simulink subsystem "PMSM_Controller"  (R2021b)
settings: Solver=VariableStepAuto  StartTime=0.0  StopTime=10.0  RelTol=1e-3
model mask{ControllerParameters=0}
  mask prompts: ControllerParameters "Controller Parameters (struct)"
undefined symbols (not defined in the file): denZC_id, denZC_iq, denZC_w, ee_sli_rtmsupport, gcbh, numZC_id, numZC_iq, numZC_w, PowSupplyParams
libraries: eeDiscretePi x3, slctrlblks x2, eeTransforms x2, eeDqVoltageLimiter x1, eePmsmCurrentReferenceGen x1, simulink x1, eePwmGeneratorTwoLevel x1
Description:
  | PMSM Controller Subsystem Reference.
  | Copyright 2021 The MathWorks, Inc.
settings Model: Creator=agonzale  LastModifiedBy=agonzale

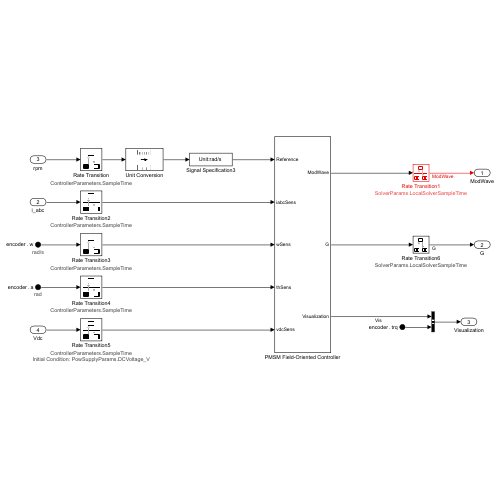
[thumbnail: Simulink's stored preview of the top-level diagram]
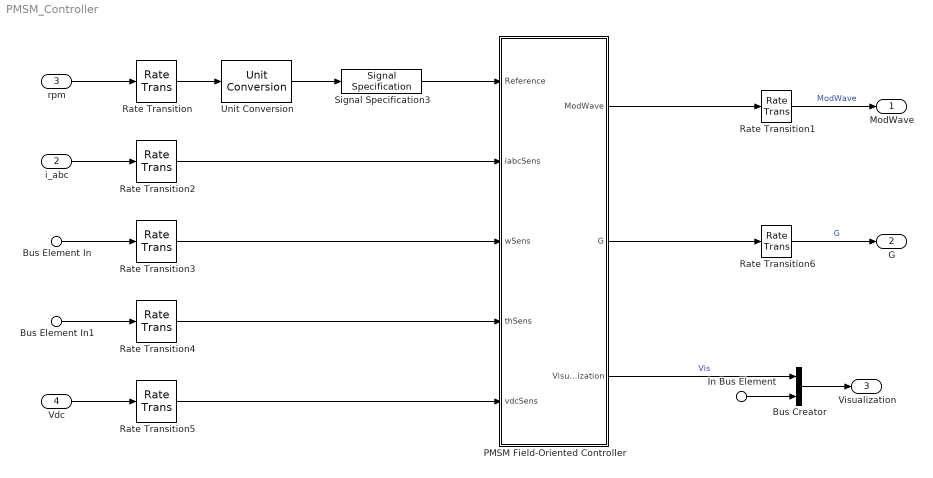
== system PMSM_Controller ==
  Bus Element In : Inport  PortName=encoder  Element=w
      settings: AttributesFormatString=%<Unit>
  Bus Element In1 : Inport  PortName=encoder  Element=a
      settings: AttributesFormatString=%<Unit>
  In Bus Element : Inport  PortName=encoder  Element=trq
  i_abc : Inport  Port=2
  rpm : Inport  Port=3  Unit=rpm
  Vdc : Inport  Port=4
  Bus Creator : BusCreator  Inputs=2
  PMSM Field-Oriented Controller : Subsystem  LoadFcn=ee_sli_rtmsupport( 'loadfcn', gcbh );  VariantControl=Estimation  mask(PMSM Field-Oriented Control){winding_type=Wye-wound, CtrlMode=Velocity control, Vnom=ControllerParameters.VdcNominal, Pmax=ControllerParameters.PowMax, Tmax=ControllerParameters.TrqMax, p=ControllerParameters.NumPolePairs, Vdc_on=ControllerParameters.InverterVdcThreshold, Ts=ControllerParameters.FundamentalSampleTime, Tsc=ControllerParameters.SampleTime, CtrlType=PI control, Kp_w=ControllerParameters.OuterLoop.PropGain, Ki_w=ControllerParameters.OuterLoop.IntegGain, Kv_w=1, Kaw_w=ControllerParameters.OuterLoop.AntiWindupIntegGain, RefType=Lookup-table based, rpmVec=ControllerParameters.OuterLoop.RpmVec, TqVec=ControllerParameters.OuterLoop.TrqRefVec, VdcVec=ControllerParameters.OuterLoop.VdcVec, PWMMode=SPWM: sinusoidal PWM, ModFactor=1, idMatrix=ControllerParameters.OuterLoop.iDrefMat, iqMatrix=ControllerParameters.OuterLoop.iQrefMat, psim=1, Ld=0.00024, Lq=0.00029, Rs=1, AxisAlignment=Q-axis, Kp_id=ControllerParameters.InnerLoop.PropGain_iD, Ki_id=ControllerParameters.InnerLoop.IntegGain_iD, Kaw_id=ControllerParameters.InnerLoop.AntiWindupIntegGain_iD, Kp_iq=ControllerParameters.InnerLoop.PropGain_iQ, Ki_iq=ControllerParameters.InnerLoop.IntegGain_iQ, Kaw_iq=ControllerParameters.InnerLoop.AntiWindupIntegGain_iQ, AxisPrio=Q-axis, ActZC=off, ActFF=off, ParamTypeFF=Constant parameters, LdFF=1, LqFF=1, psimFF=1, idVect=[-200, 0, 200], iqVect=[-200, 0, 200], LdMatrix=0.0002 * ones(3, 3), LqMatrix=0.0002 * ones(3, 3), psimMatrix=0.04 * ones(3, 3), CPWMMode=SPWM: sinusoidal PWM, SamplingMode=Natural, fsw=ControllerParameters.InverterSwitchingFrequency}
      mask prompts: winding_type "Winding type"; CtrlMode "physmod:ee:library:comments:control:eePmsmFieldOrientedControl:ControlMode_MP"; Vnom "physmod:ee:library:comments:control:eePmsmFieldOrientedControl:NominalDclinkVoltageV_MP"; Pmax "physmod:ee:library:comments:control:eePmsmFieldOrientedControl:MaximumPowerW_MP"; Tmax "physmod:ee:library:comments:control:eePmsmFieldOrientedControl:MaximumTorqueNm_MP"; p "physmod:ee:library:comments:control:eePmsmFieldOrientedControl:NumberOfRotorPolePairs_MP"; Vdc_on "physmod:ee:library:comments:control:eePmsmFieldOrientedControl:InverterDclinkVoltageThresholdV_MP"; Ts "physmod:ee:library:comments:control:eePmsmFieldOrientedControl:FundamentalSampleTimes_MP"; Tsc "physmod:ee:library:comments:control:eePmsmFieldOrientedControl:ControlSampleTimes_MP"; CtrlType "physmod:ee:library:comments:control:eePmsmFieldOrientedControl:ControlType_MP"; Kp_w "physmod:ee:library:comments:control:eePmsmFieldOrientedControl:ControllerProportionalGain_MP"; Ki_w "physmod:ee:library:comments:control:eePmsmFieldOrientedControl:ControllerIntegralGain_MP"; Kv_w "physmod:ee:library:comments:control:eePmsmFieldOrientedControl:PControllerProportionalGain_MP"; Kaw_w "physmod:ee:library:comments:control:eePmsmFieldOrientedControl:IntegralAntiwindupGain_MP"; RefType "physmod:ee:library:comments:control:eePmsmFieldOrientedControl:CurrentReferences_MP"; rpmVec "physmod:ee:library:comments:control:eePmsmFieldOrientedControl:MechanicalSpeedVectorWMechanicalrpm_MP"; TqVec "physmod:ee:library:comments:control:eePmsmFieldOrientedControl:TorqueReferenceVectorTqRefNm_MP"; VdcVec "physmod:ee:library:comments:control:eePmsmFieldOrientedControl:DClinkVoltageVectorVdcV_MP"; PWMMode "physmod:ee:library:comments:control:eePmsmCurrentReferenceGen:PWMMethod_MP"; ModFactor "physmod:ee:library:comments:control:eePmsmCurrentReferenceGen:ModulationFactor_MP"; idMatrix "physmod:ee:library:comments:control:eePmsmFieldOrientedControl:DaxisCurrentReferenceMatrixIdwMechanicalTqRefVdcA_MP"; iqMatrix "physmod:ee:library:comments:control:eePmsmFieldOrientedControl:QaxisCurrentReferenceMatrixIqwMechanicalTqRefVdcA_MP"; psim "physmod:ee:library:comments:control:eePmsmFieldOrientedControl:PermanentMagnetFluxLinkageWb_MP"; Ld "physmod:ee:library:comments:control:eePmsmFieldOrientedControl:DaxisInductanceH_MP"; Lq "physmod:ee:library:comments:control:eePmsmFieldOrientedControl:QaxisInductanceH_MP"; Rs "physmod:ee:library:comments:control:eePmsmFieldOrientedControl:StatorResistanceOhm_MP"; AxisAlignment "physmod:ee:library:comments:control:eePmsmFieldOrientedControl:PhaseaAxisAlignment_MP"; Kp_id "physmod:ee:library:comments:control:eePmsmFieldOrientedControl:DaxisCurrentProportionalGain_MP"; Ki_id "physmod:ee:library:comments:control:eePmsmFieldOrientedControl:DaxisCurrentIntegralGain_MP"; Kaw_id "physmod:ee:library:comments:control:eePmsmFieldOrientedControl:DaxisCurrentAntiwindupGain_MP"; Kp_iq "physmod:ee:library:comments:control:eePmsmFieldOrientedControl:QaxisCurrentProportionalGain_MP"; Ki_iq "physmod:ee:library:comments:control:eePmsmFieldOrientedControl:QaxisCurrentIntegralGain_MP"; Kaw_iq "physmod:ee:library:comments:control:eePmsmFieldOrientedControl:QaxisCurrentAntiwindupGain_MP"; AxisPrio "physmod:ee:library:comments:control:eePmsmFieldOrientedControl:AxisPrioritization_MP"; ActZC "physmod:ee:library:comments:control:eePmsmFieldOrientedControl:EnableZeroCancellation_MP"; ActFF "physmod:ee:library:comments:control:eePmsmFieldOrientedControl:EnablePrecontrolVoltage_MP"; ParamTypeFF "physmod:ee:library:comments:control:eePmsmFieldOrientedControl:MachineParameters_MP"; LdFF "physmod:ee:library:comments:control:eePmsmFieldOrientedControl:DaxisInductanceForFeedforwardPrecontrolH_MP"; LqFF "physmod:ee:library:comments:control:eePmsmFieldOrientedControl:QaxisInductanceForFeedforwardPrecontrolH_MP"; psimFF "physmod:ee:library:comments:control:eePmsmFieldOrientedControl:PermanentMagnetFluxLinkageForFeedforwardPrecontrolWb_MP"; idVect "physmod:ee:library:comments:control:eePmsmFieldOrientedControl:DaxisCurrentVectorIdA_MP"; iqVect "physmod:ee:library:comments:control:eePmsmFieldOrientedControl:QaxisCurrentVectorIqA_MP"; LdMatrix "physmod:ee:library:comments:control:eePmsmFieldOrientedControl:LdMatrixLdidiqH_MP"; LqMatrix "physmod:ee:library:comments:control:eePmsmFieldOrientedControl:LqMatrixLqidiqH_MP"; psimMatrix "physmod:ee:library:comments:control:eePmsmFieldOrientedControl:PermanentMagnetFluxLinkageMatrixPMidiqWb_MP"; CPWMMode "physmod:ee:library:comments:control:eePmsmFieldOrientedControl:PWMMethod_MP"; SamplingMode "physmod:ee:library:comments:control:eePmsmFieldOrientedControl:SamplingMode_MP"; fsw "physmod:ee:library:comments:control:eePmsmFieldOrientedControl:SwitchingFrequencyHz_MP"
      mask help: physmod:ee:library:comments:control:eePmsmFieldOrientedControl:PMSMFieldOrientedControl_MD
      mask init:
      | if ParamTypeFF == 1
      |     idVect = [-200, 200];
      |     iqVect = [-200, 200];
      |     LdMatrix = LdFF*ones(2, 2);
      |     LqMatrix = LqFF*ones(2, 2);
      |     psimMatrix = psimFF*ones(2, 2);
      | end
      | 
      | switch winding_type
      |     case 1
      |         theta_offset = 0;
      |     case 2
      |         theta_offset = -(120/p)*pi/180;
      |     otherwise
      |         theta_offset = 0;
      | end
      | 
      | switch CPWMMode
      |     case 'SPWM: sinusoidal PWM'
      |         set_param(gcb,'PWMMode','SPWM: sinusoidal PWM');
      |     case 'SVM: space vector modulation'
      |         set_param(gcb,'PWMMode','SVM: space vector modulation')
      | end
      settings: CopyFcn=ee_sli_rtmsupport( 'copyfcn', gcbh );  DeleteFcn=ee_sli_rtmsupport( 'deletefcn', gcbh );  ModelCloseFcn=ee_sli_rtmsupport( 'modelclosefcn', gcbh );  PostSaveFcn=ee_sli_rtmsupport( 'postsavefcn', gcbh );  PreCopyFcn=ee_sli_rtmsupport( 'precopyfcn', gcbh );  OpenFcn=ee_sli_rtmsupport( 'openfcn', gcbh );  CloseFcn=ee_sli_rtmsupport( 'closefcn', gcbh );  PreDeleteFcn=ee_sli_rtmsupport( 'predeletefcn', gcbh );
      mask Help: web(nesl_help(gcbh))
      mask TypeOptions winding_type: Wye-wound | Delta-wound
      mask TypeOptions CtrlMode: physmod:ee:library:comments:control:eePmsmFieldOrientedControl:VelocityControl_PV | physmod:ee:library:comments:control:eePmsmFieldOrientedControl:TorqueControl_PV
      mask Callback CtrlMode: ee.mask.callbackPopupPmsmFoc(gcb);
      mask TypeOptions Vnom:
      | Outer loop control/PMSM Current Reference
      | Generator/Vnom
      mask TypeOptions Pmax:
      | Outer loop control/PMSM Current Reference
      | Generator/Pmax
      mask TypeOptions Tmax:
      | Outer loop control/PMSM Current Reference
      | Generator/Tmax
      mask TypeOptions CtrlType: Outer loop control/Velocity Controller/CtrlType
      mask Callback CtrlType: ee.mask.callbackPopupPmsmFoc(gcb);
      mask TypeOptions Kp_w: Outer loop control/Velocity Controller/Kp_w
      mask TypeOptions Ki_w: Outer loop control/Velocity Controller/Ki_w
      mask TypeOptions Kv_w: Outer loop control/Velocity Controller/Kv_w
      mask TypeOptions Kaw_w: Outer loop control/Velocity Controller/Kaw_w
      mask TypeOptions RefType:
      | Outer loop control/PMSM Current Reference
      | Generator/RefType
      mask Callback RefType: ee.mask.callbackPopupPmsmFoc(gcb);
      mask TypeOptions rpmVec:
      | Outer loop control/PMSM Current Reference
      | Generator/rpmVec
      mask TypeOptions TqVec:
      | Outer loop control/PMSM Current Reference
      | Generator/TqVec
      mask TypeOptions VdcVec:
      | Outer loop control/PMSM Current Reference
      | Generator/VdcVec
      mask TypeOptions PWMMode:
      | Outer loop control/PMSM Current Reference
      | Generator/PWMMode
      mask TypeOptions ModFactor:
      | Outer loop control/PMSM Current Reference
      | Generator/ModFactor
      mask TypeOptions idMatrix:
      | Outer loop control/PMSM Current Reference
      | Generator/idMatrix
      mask TypeOptions iqMatrix:
      | Outer loop control/PMSM Current Reference
      | Generator/iqMatrix
      mask TypeOptions psim:
      | Outer loop control/PMSM Current Reference
      | Generator/psim
      mask TypeOptions Ld:
      | Outer loop control/PMSM Current Reference
      | Generator/Ld
      mask TypeOptions Lq:
      | Outer loop control/PMSM Current Reference
      | Generator/Lq
      mask TypeOptions Rs:
      | Outer loop control/PMSM Current Reference
      | Generator/Rs
      mask TypeOptions AxisAlignment: Inner loop control/Park Transform/AxisAlignment
      mask TypeOptions Kp_id:
      | Inner loop control/PMSM Current Controller
      | with Pre-Control/Kp_id
      mask TypeOptions Ki_id:
      | Inner loop control/PMSM Current Controller
      | with Pre-Control/Ki_id
      mask TypeOptions Kaw_id:
      | Inner loop control/PMSM Current Controller
      | with Pre-Control/Kaw_id
      mask TypeOptions Kp_iq:
      | Inner loop control/PMSM Current Controller
      | with Pre-Control/Kp_iq
      mask TypeOptions Ki_iq:
      | Inner loop control/PMSM Current Controller
      | with Pre-Control/Ki_iq
      mask TypeOptions Kaw_iq:
      | Inner loop control/PMSM Current Controller
      | with Pre-Control/Kaw_iq
      mask TypeOptions AxisPrio:
      | Inner loop control/PMSM Current Controller
      | with Pre-Control/AxisPrio
      mask TypeOptions ActZC:
      | Inner loop control/PMSM Current Controller
      | with Pre-Control/ActZC
      mask TypeOptions ActFF:
      | Inner loop control/PMSM Current Controller
      | with Pre-Control/ActFF
      mask Callback ActFF: ee.mask.callbackPopupPmsmFoc(gcb);
      mask TypeOptions ParamTypeFF: physmod:ee:library:comments:control:eePmsmFieldOrientedControl:ConstantParameters_PV | physmod:ee:library:comments:control:eePmsmFieldOrientedControl:LookupTableBasedParameters_PV
      mask Callback ParamTypeFF: ee.mask.callbackPopupPmsmFoc(gcb);
      mask TypeOptions idVect:
      | Inner loop control/PMSM Current Controller
      | with Pre-Control/idVect
      mask TypeOptions iqVect:
      | Inner loop control/PMSM Current Controller
      | with Pre-Control/iqVect
      mask TypeOptions LdMatrix:
      | Inner loop control/PMSM Current Controller
      | with Pre-Control/LdMatrix
      mask TypeOptions LqMatrix:
      | Inner loop control/PMSM Current Controller
      | with Pre-Control/LqMatrix
      mask TypeOptions psimMatrix:
      | Inner loop control/PMSM Current Controller
      | with Pre-Control/psimMatrix
      mask TypeOptions CPWMMode:
      | PWM/PWM Generator
      | (Three-phase, Two-level)/PWM/CPWMMode
      mask TypeOptions SamplingMode:
      | PWM/PWM Generator
      | (Three-phase, Two-level)/PWM/SamplingMode
      mask DialogControl Container4 Prompt: physmod:ee:library:comments:control:eePmsmFieldOrientedControl:tab_General
      mask DialogControl CtrlMode Prompt: Control mode
      mask DialogControl Vnom Prompt: Nominal dc-link voltage (V)
      mask DialogControl Pmax Prompt: Maximum power (W)
      mask DialogControl Tmax Prompt: Maximum torque (N*m)
      mask DialogControl p Prompt: Number of rotor pole pairs
      mask DialogControl Vdc_on Prompt: Inverter dc-link voltage threshold (V)
      mask DialogControl Ts Prompt: Fundamental sample time (s)
      mask DialogControl Tsc Prompt: Control sample time (s)
      mask DialogControl Container7 Prompt: physmod:ee:library:comments:control:eePmsmFieldOrientedControl:tab_OuterLoop
      mask DialogControl CtrlType Prompt: Control type
      mask DialogControl Kp_w Prompt: Controller proportional gain
      mask DialogControl Ki_w Prompt: Controller integral gain
      mask DialogControl Kv_w Prompt: P controller proportional gain
      mask DialogControl Kaw_w Prompt: Integral anti-windup gain
      mask DialogControl RefType Prompt: Current references
      mask DialogControl rpmVec Prompt: Mechanical speed vector, wMechanical (rpm)
      mask DialogControl TqVec Prompt: Torque reference vector, TqRef (N*m)
      mask DialogControl VdcVec Prompt: DC-link voltage vector, Vdc (V)
      mask DialogControl PWMMode Prompt: PWM method
      mask DialogControl ModFactor Prompt: Modulation factor
      mask DialogControl idMatrix Prompt: D-axis current reference matrix, id(wMechanical,TqRef,Vdc), (A)
      mask DialogControl iqMatrix Prompt: Q-axis current reference matrix, iq(wMechanical,TqRef,Vdc), (A)
      mask DialogControl psim Prompt: Permanent magnet flux linkage (Wb)
      mask DialogControl Ld Prompt: D-axis inductance (H)
      mask DialogControl Lq Prompt: Q-axis inductance (H)
      mask DialogControl Rs Prompt: Stator resistance (Ohm)
      mask DialogControl Container8 Prompt: physmod:ee:library:comments:control:eePmsmFieldOrientedControl:tab_InnerLoop
      mask DialogControl AxisAlignment Prompt: Phase-a axis alignment
      mask DialogControl Kp_id Prompt: D-axis current proportional gain
      mask DialogControl Ki_id Prompt: D-axis current integral gain
      mask DialogControl Kaw_id Prompt: D-axis current anti-windup gain
      mask DialogControl Kp_iq Prompt: Q-axis current proportional gain
      mask DialogControl Ki_iq Prompt: Q-axis current integral gain
      mask DialogControl Kaw_iq Prompt: Q-axis current anti-windup gain
      mask DialogControl AxisPrio Prompt: Axis prioritization
      mask DialogControl ActZC Prompt: Enable zero cancellation
      mask DialogControl ActFF Prompt: Enable pre-control voltage
      mask DialogControl ParamTypeFF Prompt: Machine parameters
      mask DialogControl LdFF Prompt: D-axis inductance for feed-forward pre-control (H)
      mask DialogControl LqFF Prompt: Q-axis inductance for feed-forward pre-control (H)
      mask DialogControl psimFF Prompt: Permanent magnet flux linkage for feed-forward pre-control (Wb)
      mask DialogControl idVect Prompt: D-axis current vector, id (A)
      mask DialogControl iqVect Prompt: Q-axis current vector, iq (A)
      mask DialogControl LdMatrix Prompt: Ld matrix, Ld(id,iq), (H)
      mask DialogControl LqMatrix Prompt: Lq matrix, Lq(id,iq), (H)
      mask DialogControl psimMatrix Prompt: Permanent magnet flux linkage matrix, PM(id,iq), (Wb)
      mask DialogControl Container9 Prompt: physmod:ee:library:comments:control:eePmsmFieldOrientedControl:tab_PWM
      mask DialogControl CPWMMode Prompt: PWM method
      mask DialogControl SamplingMode Prompt: Sampling mode
      mask DialogControl fsw Prompt: Switching frequency (Hz)
  Rate Transition{,2..4} (4 alike) : RateTransition  OutPortSampleTime=ControllerParameters.SampleTime
      settings: AttributesFormatString=%<OutPortSampleTime>
  Rate Transition1 : RateTransition  OutPortSampleTime=SolverParams.LocalSolverSampleTime
      settings: AttributesFormatString=%<OutPortSampleTime>
  Rate Transition5 : RateTransition  InitialCondition=PowSupplyParams.DCVoltage_V  OutPortSampleTime=ControllerParameters.SampleTime
      settings: AttributesFormatString=|
      | %<OutPortSampleTime>
      | Initial Condition: %<InitialCondition>
  Rate Transition6 : RateTransition  OutPortSampleTime=SolverParams.LocalSolverSampleTime
      settings: AttributesFormatString=%<OutPortSampleTime>
  Signal Specification3 : SignalSpecification  Unit=rad/s
  Unit Conversion : UnitConversion
  ModWave : Outport  VectorParamsAs1DForOutWhenUnconnected=off
  G : Outport  Port=2  VectorParamsAs1DForOutWhenUnconnected=off
  Visualization : Outport  Port=3  VectorParamsAs1DForOutWhenUnconnected=off
  wires:
  Vdc/1 -> Rate Transition5/1
  PMSM Field-Oriented Controller/1(ModWave) -> Rate Transition1/1
  Signal Specification3/1 -> PMSM Field-Oriented Controller/1(Reference)
  Unit Conversion/1 -> Signal Specification3/1
  Rate Transition1/1 -> ModWave/1  "ModWave"
  rpm/1 -> Rate Transition/1
  Rate Transition/1 -> Unit Conversion/1
  i_abc/1 -> Rate Transition2/1
  Rate Transition2/1 -> PMSM Field-Oriented Controller/2(iabcSens)
  Bus Element In/1 -> Rate Transition3/1
  Rate Transition3/1 -> PMSM Field-Oriented Controller/3(wSens)
  Bus Element In1/1 -> Rate Transition4/1
  Rate Transition4/1 -> PMSM Field-Oriented Controller/4(thSens)
  Rate Transition5/1 -> PMSM Field-Oriented Controller/5(vdcSens)
  Rate Transition6/1 -> G/1  "G"
  PMSM Field-Oriented Controller/2(G) -> Rate Transition6/1
  PMSM Field-Oriented Controller/3(Visualization) -> Bus Creator/1  "Vis"
  In Bus Element/1 -> Bus Creator/2
  Bus Creator/1 -> Visualization/1

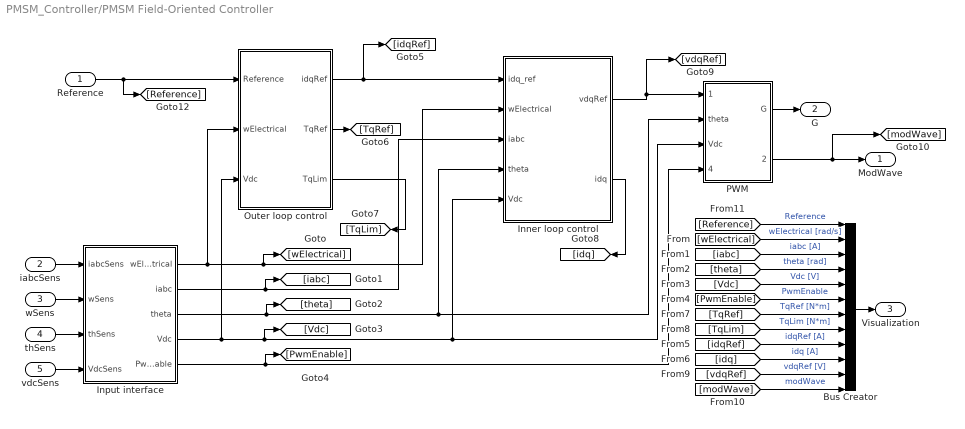
== system PMSM_Controller/PMSM Field-Oriented Controller ==
  Reference : Inport  SampleTime=Tsc
  iabcSens : Inport  Port=2  SampleTime=Tsc
  wSens : Inport  Port=3  SampleTime=Tsc
  thSens : Inport  Port=4  SampleTime=Tsc
  vdcSens : Inport  Port=5  SampleTime=Tsc
  Bus Creator : BusCreator  Inputs=12
  Inner loop control : Subsystem  VariantControl=Estimation
  Input interface : Subsystem
  Outer loop control : Subsystem  VariantControl=Estimation
  PWM : Subsystem
  ModWave : Outport  VectorParamsAs1DForOutWhenUnconnected=off
  G : Outport  Port=2  VectorParamsAs1DForOutWhenUnconnected=off
  Visualization : Outport  Port=3  VectorParamsAs1DForOutWhenUnconnected=off
  wires:
  PWM/1(G) -> G/1
  PWM/2(ModWave) -> ModWave/1, [modWave]
  Input interface/3(theta) -> [theta], PWM/2(theta), Inner loop control/4(theta)
  Input interface/2(iabc) -> [iabc], Inner loop control/3(iabc)
  Outer loop control/1(idqRef) -> Inner loop control/1(idq_ref), [idqRef]
  iabcSens/1 -> Input interface/1(iabcSens)
  wSens/1 -> Input interface/2(wSens)
  thSens/1 -> Input interface/3(thSens)
  vdcSens/1 -> Input interface/4(VdcSens)
  Reference/1 -> [Reference], Outer loop control/1(Reference)
  Input interface/4(Vdc) -> Outer loop control/3(Vdc), [Vdc], PWM/3(Vdc), Inner loop control/5(Vdc)
  Input interface/1(wElectrical) -> Outer loop control/2(wElectrical), [wElectrical], Inner loop control/2(wElectrical)
  Inner loop control/1(vdqRef) -> [vdqRef], PWM/1(vdqRef)
  Input interface/5(PwmEnable) -> [PwmEnable], PWM/4(PwmEnable)
  Bus Creator/1 -> Visualization/1
  Outer loop control/2(TqRef) -> [TqRef]
  Outer loop control/3(TqLim) -> [TqLim]
  Inner loop control/2(idq) -> [idq]
  [Reference] -> Bus Creator/1  "Reference"
  [wElectrical] -> Bus Creator/2  "wElectrical [rad/s]"
  [iabc] -> Bus Creator/3  "iabc [A]"
  [theta] -> Bus Creator/4  "theta [rad]"
  [Vdc] -> Bus Creator/5  "Vdc [V]"
  [PwmEnable] -> Bus Creator/6  "PwmEnable"
  [TqRef] -> Bus Creator/7  "TqRef [N*m]"
  [TqLim] -> Bus Creator/8  "TqLim [N*m]"
  [idqRef] -> Bus Creator/9  "idqRef [A]"
  [idq] -> Bus Creator/10  "idq [A]"
  [vdqRef] -> Bus Creator/11  "vdqRef [V]"
  [modWave] -> Bus Creator/12  "modWave"

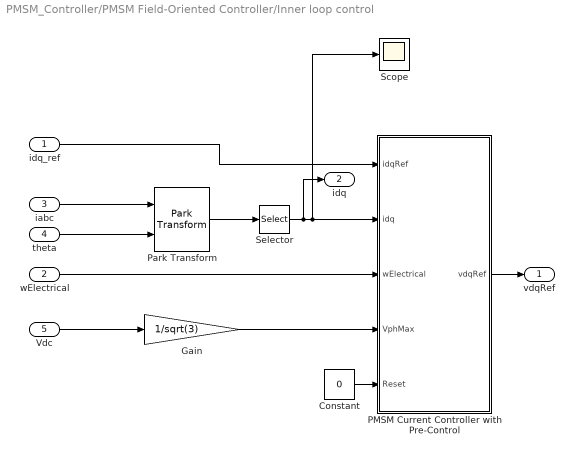
== system PMSM_Controller/PMSM Field-Oriented Controller/Inner loop control ==
  idq_ref : Inport
  wElectrical : Inport  Port=2
  iabc : Inport  Port=3
  theta : Inport  Port=4
  Vdc : Inport  Port=5
  Constant : Constant  Value=0  SampleTime=-1
  Gain : Gain  Gain=1/sqrt(3)
  PMSM Current Controller with Pre-Control : Subsystem  LoadFcn=ee_sli_rtmsupport( 'loadfcn', gcbh );  mask(PMSM Current Controller with Pre-Control){Kp_id=Kp_id, Ki_id=Ki_id, Kaw_id=Kaw_id, Kp_iq=Kp_iq, Ki_iq=Ki_iq, Kaw_iq=Kaw_iq, Ts=Tsc, Tsd=0.001, AxisPrio=Q-axis, ActZC=off, ActFF=off, idVect=idVect, iqVect=iqVect, LdMatrix=LdMatrix, LqMatrix=LqMatrix, psimMatrix=psimMatrix}
      mask prompts: Kp_id "physmod:ee:library:comments:control:eePmsmCurrentController:DaxisCurrentProportionalGain_MP"; Ki_id "physmod:ee:library:comments:control:eePmsmCurrentController:DaxisCurrentIntegralGain_MP"; Kaw_id "physmod:ee:library:comments:control:eePmsmCurrentController:DaxisCurrentAntiwindupGain_MP"; Kp_iq "physmod:ee:library:comments:control:eePmsmCurrentController:QaxisCurrentProportionalGain_MP"; Ki_iq "physmod:ee:library:comments:control:eePmsmCurrentController:QaxisCurrentIntegralGain_MP"; Kaw_iq "physmod:ee:library:comments:control:eePmsmCurrentController:QaxisCurrentAntiwindupGain_MP"; Ts "physmod:ee:library:comments:control:eePmsmCurrentController:SampleTime1ForInherited_MP"; Tsd "physmod:ee:library:comments:control:eePmsmCurrentController:DiscretizationSampleTime_MP"; AxisPrio "physmod:ee:library:comments:control:eePmsmCurrentController:AxisPrioritization_MP"; ActZC "physmod:ee:library:comments:control:eePmsmCurrentController:EnableZeroCancellation_MP"; ActFF "physmod:ee:library:comments:control:eePmsmCurrentController:EnablePrecontrolVoltage_MP"; idVect "physmod:ee:library:comments:control:eePmsmCurrentController:DaxisCurrentVectorIdA_MP"; iqVect "physmod:ee:library:comments:control:eePmsmCurrentController:QaxisCurrentVectorIqA_MP"; LdMatrix "physmod:ee:library:comments:control:eePmsmCurrentController:LdMatrixLdidiqH_MP"; LqMatrix "physmod:ee:library:comments:control:eePmsmCurrentController:LqMatrixLqidiqH_MP"; psimMatrix "physmod:ee:library:comments:control:eePmsmCurrentController:PermanentMagnetFluxLinkageMatrixPMidiqWb_MP"
      mask help: physmod:ee:library:comments:control:eePmsmCurrentController:PMSMCurrentControllerWithPreControl_MD
      mask init:
      | [Tsd, numZC_id, denZC_id, numZC_iq, denZC_iq] = ee.mask.initializePmsmCurrentController(ActZC,Ts,Tsd,Kp_id,Ki_id,Kp_iq,Ki_iq);
      | 
      | if length(idVect) < 2            
      | 	error(message('physmod:simscape:compiler:patterns:checks:LengthGreaterThanOrEqual',getString(message('physmod:ee:library:comments:control:eePmsmCurrentController:DaxisCurrentVectorIdA_MP')), '2'));            
      | end
      | if ~all(diff(idVect) > 0)            
      | 	error(message('physmod:simscape:compiler:patterns:checks:StrictlyAscendingVec',getString(message('physmod:ee:library:comments:control:eePmsmCurrentController:DaxisCurrentVectorIdA_MP'))));            
      | end
      | if length(iqVect) < 2            
      | 	error(message('physmod:simscape:compiler:patterns:checks:LengthGreaterThanOrEqual',getString(message('physmod:ee:library:comments:control:eePmsmCurrentController:QaxisCurrentVectorIqA_MP')), '2'));            
      | end
      | if ~all(diff(iqVect) > 0)            
      | 	error(message('physmod:simscape:compiler:patterns:checks:StrictlyAscendingVec',getString(message('physmod:ee:library:comments:control:eePmsmCurrentController:QaxisCurrentVectorIqA_MP'))));            
      | end
      | if ~all(size(LdMatrix) == [length(idVect), length(iqVect)])            
      | 	error(message('physmod:simscape:compiler:patterns:checks:Size2DEqual',getString(message('physmod:ee:library:comments:control:eePmsmCurrentController:LdMatrixLdidiqH_MP')), getString(message('physmod:ee:library:comments:control:eePmsmCurrentController:DaxisCurrentVectorIdA_MP')), getString(message('physmod:ee:library:comments:control:eePmsmCurrentController:QaxisCurrentVectorIqA_MP'))));            
      | end
      | if ~all(size(LqMatrix) == [length(idVect), length(iqVect)])            
      | 	error(message('physmod:simscape:compiler:patterns:checks:Size2DEqual',getString(message('physmod:ee:library:comments:control:eePmsmCurrentController:LqMatrixLqidiqH_MP')), getString(message('physmod:ee:library:comments:control:eePmsmCurrentController:DaxisCurrentVectorIdA_MP')), getString(message('physmod:ee:library:comments:control:eePmsmCurrentController:QaxisCurrentVectorIqA_MP'))));            
      | end
      | if ~all(size(psimMatrix) == [length(idVect), length(iqVect)])            
      | 	error(message('physmod:simscape:compiler:patterns:checks:Size2DEqual',getString(message('physmod:ee:library:comments:control:eePmsmCurrentController:PermanentMagnetFluxLinkageMatrixPMidiqWb_MP')), getString(message('physmod:ee:library:comments:control:eePmsmCurrentController:DaxisCurrentVectorIdA_MP')), getString(message('physmod:ee:library:comments:control:eePmsmCurrentController:QaxisCurrentVectorIqA_MP'))));            
      | end
      settings: CopyFcn=ee_sli_rtmsupport( 'copyfcn', gcbh );  DeleteFcn=ee_sli_rtmsupport( 'deletefcn', gcbh );  ModelCloseFcn=ee_sli_rtmsupport( 'modelclosefcn', gcbh );  PostSaveFcn=ee_sli_rtmsupport( 'postsavefcn', gcbh );  PreCopyFcn=ee_sli_rtmsupport( 'precopyfcn', gcbh );  OpenFcn=ee_sli_rtmsupport( 'openfcn', gcbh );  CloseFcn=ee_sli_rtmsupport( 'closefcn', gcbh );  PreDeleteFcn=ee_sli_rtmsupport( 'predeletefcn', gcbh );
      mask Help: web(nesl_help(gcbh))
      mask Callback Ts: ee.mask.callbackZeroCancellation(gcb);
      mask TypeOptions AxisPrio: d-q Voltage Limiter/AxisPrio
      mask Callback ActZC: ee.mask.callbackZeroCancellation(gcb);
      mask DialogControl Container3 Prompt: physmod:ee:library:comments:control:eePmsmCurrentController:tab_ControlParameters
      mask DialogControl Kp_id Prompt: D-axis current proportional gain
      mask DialogControl Ki_id Prompt: D-axis current integral gain
      mask DialogControl Kaw_id Prompt: D-axis current anti-windup gain
      mask DialogControl Kp_iq Prompt: Q-axis current proportional gain
      mask DialogControl Ki_iq Prompt: Q-axis current integral gain
      mask DialogControl Kaw_iq Prompt: Q-axis current anti-windup gain
      mask DialogControl Ts Prompt: Sample time (-1 for inherited)
      mask DialogControl Tsd Prompt: Discretization sample time
      mask DialogControl AxisPrio Prompt: Axis prioritization
      mask DialogControl ActZC Prompt: Enable zero cancellation
      mask DialogControl ActFF Prompt: Enable pre-control voltage
      mask DialogControl Container4 Prompt: physmod:ee:library:comments:control:eePmsmCurrentController:tab_PreControlParameters
      mask DialogControl idVect Prompt: D-axis current vector, id (A)
      mask DialogControl iqVect Prompt: Q-axis current vector, iq (A)
      mask DialogControl LdMatrix Prompt: Ld matrix, Ld(id,iq), (H)
      mask DialogControl LqMatrix Prompt: Lq matrix, Lq(id,iq), (H)
      mask DialogControl psimMatrix Prompt: Permanent magnet flux linkage matrix, PM(id,iq), (Wb)
  Park Transform : eeTransforms/Park Transform  AxisAlignment=Q-axis  PowerInvariant=off
  Scope : Scope
  Selector : Selector  InputPortWidth=3  IndexOptions=Index vector (dialog)  Indices=[1 2]  OutputSizes=1
  vdqRef : Outport  VectorParamsAs1DForOutWhenUnconnected=off
  idq : Outport  Port=2  VectorParamsAs1DForOutWhenUnconnected=off
  wires:
  idq_ref/1 -> PMSM Current Controller with Pre-Control/1(idqRef)
  Constant/1 -> PMSM Current Controller with Pre-Control/5(Reset)
  Selector/1 -> PMSM Current Controller with Pre-Control/2(idq), Scope/1, idq/1
  Gain/1 -> PMSM Current Controller with Pre-Control/4(VphMax)
  Park Transform/1 -> Selector/1
  iabc/1 -> Park Transform/1
  theta/1 -> Park Transform/2
  wElectrical/1 -> PMSM Current Controller with Pre-Control/3(wElectrical)
  Vdc/1 -> Gain/1
  PMSM Current Controller with Pre-Control/1(vdqRef) -> vdqRef/1

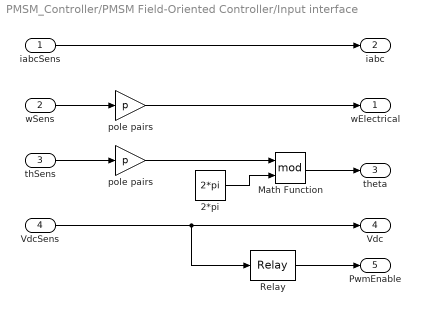
== system PMSM_Controller/PMSM Field-Oriented Controller/Input interface ==
  iabcSens : Inport
  wSens : Inport  Port=2
  thSens : Inport  Port=3
  VdcSens : Inport  Port=4
  2*pi : Constant  Value=2*pi  SampleTime=Tsc
  Math Function : Math  Operator=mod  SignedPower=on  SaturateOnIntegerOverflow=on
  Relay : Relay  OnSwitchValue=Vdc_on  OffSwitchValue=0.5*Vdc_on
  pole pairs : Gain  Gain=p
  "pole pairs " : Gain  Gain=p
  wElectrical : Outport  VectorParamsAs1DForOutWhenUnconnected=off
  iabc : Outport  Port=2  VectorParamsAs1DForOutWhenUnconnected=off
  theta : Outport  Port=3  VectorParamsAs1DForOutWhenUnconnected=off
  Vdc : Outport  Port=4  VectorParamsAs1DForOutWhenUnconnected=off
  PwmEnable : Outport  Port=5  VectorParamsAs1DForOutWhenUnconnected=off
  wires:
  pole pairs/1 -> wElectrical/1
  thSens/1 -> "pole pairs "/1
  wSens/1 -> pole pairs/1
  iabcSens/1 -> iabc/1
  "pole pairs "/1 -> Math Function/1
  2*pi/1 -> Math Function/2
  Math Function/1 -> theta/1
  Relay/1 -> PwmEnable/1
  VdcSens/1 -> Relay/1, Vdc/1

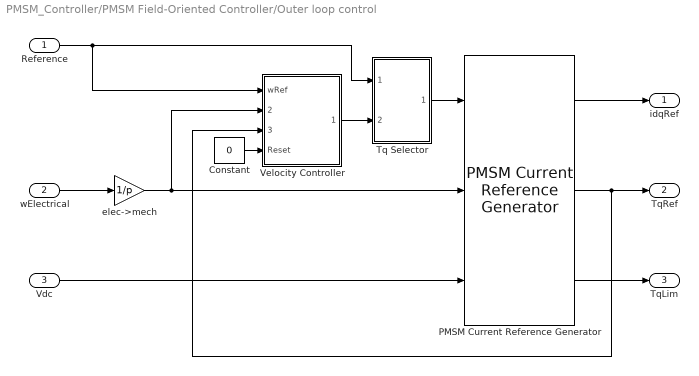
== system PMSM_Controller/PMSM Field-Oriented Controller/Outer loop control ==
  Reference : Inport
  wElectrical : Inport  Port=2
  Vdc : Inport  Port=3
  Constant : Constant  Value=0  SampleTime=-1
  PMSM Current Reference Generator : eePmsmCurrentReferenceGen/PMSM Current Reference Generator  Vnom=Vnom  Pmax=Pmax  Tmax=Tmax  Ts=Tsc  RefType=Lookup-table based  rpmVec=rpmVec  TqVec=TqVec  VdcVec=VdcVec  PWMMode=SPWM: sinusoidal PWM  ModFactor=ModFactor  idMatrix=idMatrix  iqMatrix=iqMatrix  p=p  psim=psim  Ld=Ld  Lq=Lq  Rs=Rs  RefExpEnable=0
      settings: SourceProductBaseCode=PS
  Tq Selector : Subsystem
  Velocity Controller : Subsystem  LoadFcn=ee_sli_rtmsupport( 'loadfcn', gcbh );  mask(Velocity Controller){CtrlType=PI control, Kp_w=Kp_w, Ki_w=Ki_w, Kv_w=Kv_w, Kaw_w=Kaw_w, Ts=Tsc, Tsd=0.001, ActZC=off}
      mask prompts: CtrlType "physmod:ee:library:comments:control:eeVelocityController:ControlType_MP"; Kp_w "physmod:ee:library:comments:control:eeVelocityController:ControllerProportionalGain_MP"; Ki_w "physmod:ee:library:comments:control:eeVelocityController:ControllerIntegralGain_MP"; Kv_w "physmod:ee:library:comments:control:eeVelocityController:PControllerProportionalGain_MP"; Kaw_w "physmod:ee:library:comments:control:eeVelocityController:IntegralAntiwindupGain_MP"; Ts "physmod:ee:library:comments:control:eeVelocityController:SampleTime1ForInherited_MP"; Tsd "physmod:ee:library:comments:control:eeVelocityController:DiscretizationSampleTime_MP"; ActZC "physmod:ee:library:comments:control:eeVelocityController:EnableZerocancellation_MP"
      mask help: physmod:ee:library:comments:control:eeVelocityController:VelocityController_MD
      mask init:
      | [Ki_w, Kaw_w, Tsd, numZC_w, denZC_w] = ee.mask.initializeVelocityController(CtrlType,Kp_w,Ki_w,Kaw_w,ActZC,Tsd,Ts);
      settings: CopyFcn=ee_sli_rtmsupport( 'copyfcn', gcbh );  DeleteFcn=ee_sli_rtmsupport( 'deletefcn', gcbh );  ModelCloseFcn=ee_sli_rtmsupport( 'modelclosefcn', gcbh );  PostSaveFcn=ee_sli_rtmsupport( 'postsavefcn', gcbh );  PreCopyFcn=ee_sli_rtmsupport( 'precopyfcn', gcbh );  OpenFcn=ee_sli_rtmsupport( 'openfcn', gcbh );  CloseFcn=ee_sli_rtmsupport( 'closefcn', gcbh );  PreDeleteFcn=ee_sli_rtmsupport( 'predeletefcn', gcbh );
      mask Help: web(nesl_help(gcbh))
      mask TypeOptions CtrlType: physmod:ee:library:comments:control:eeVelocityController:PIControl_PV | physmod:ee:library:comments:control:eeVelocityController:PControl_PV | physmod:ee:library:comments:control:eeVelocityController:P0x2DPIControl_PV
      mask Callback CtrlType: ee.mask.callbackPopupVelocityControl(gcb);
      mask Callback Ts: ee.mask.callbackZeroCancellation(gcb);
      mask Callback ActZC: ee.mask.callbackZeroCancellation(gcb);
      mask DialogControl Container1 Prompt: physmod:ee:library:comments:control:eeVelocityController:tab_ControlParameters
      mask DialogControl CtrlType Prompt: Control type
      mask DialogControl Kp_w Prompt: Controller proportional gain
      mask DialogControl Ki_w Prompt: Controller integral gain
      mask DialogControl Kv_w Prompt: P controller proportional gain
      mask DialogControl Kaw_w Prompt: Integral anti-windup gain
      mask DialogControl Ts Prompt: Sample time (-1 for inherited)
      mask DialogControl Tsd Prompt: Discretization sample time
      mask DialogControl ActZC Prompt: Enable zero-cancellation
  elec->mech : Gain  Gain=1/p
  idqRef : Outport  VectorParamsAs1DForOutWhenUnconnected=off
  TqRef : Outport  Port=2  VectorParamsAs1DForOutWhenUnconnected=off
  TqLim : Outport  Port=3  VectorParamsAs1DForOutWhenUnconnected=off
  wires:
  Velocity Controller/1(TqRefUnsat) -> Tq Selector/2(TqRefUnsat)
  Tq Selector/1(TqRef) -> PMSM Current Reference Generator/1
  Constant/1 -> Velocity Controller/4(Reset)
  elec->mech/1 -> Velocity Controller/2(wMechanical), PMSM Current Reference Generator/2
  PMSM Current Reference Generator/3 -> TqLim/1
  PMSM Current Reference Generator/2 -> TqRef/1, Velocity Controller/3(TqRefSat)
  PMSM Current Reference Generator/1 -> idqRef/1
  Vdc/1 -> PMSM Current Reference Generator/3
  wElectrical/1 -> elec->mech/1
  Reference/1 -> Tq Selector/1(Reference), Velocity Controller/1(wRef)

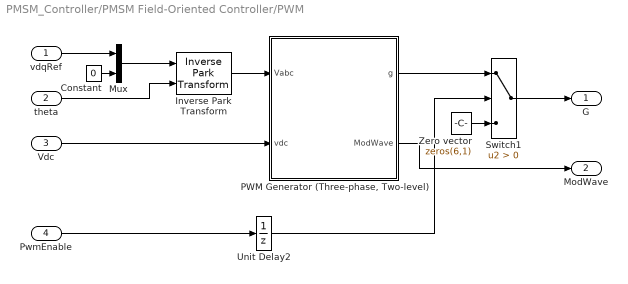
== system PMSM_Controller/PMSM Field-Oriented Controller/PWM ==
  vdqRef : Inport
  theta : Inport  Port=2
  Vdc : Inport  Port=3
  PwmEnable : Inport  Port=4
  Constant : Constant  Value=0  SampleTime=Tsc
  Inverse Park Transform : eeTransforms/Inverse Park Transform  AxisAlignment=Q-axis  PowerInvariant=off
  Mux : Mux  Inputs=2
  "PWM Generator (Three-phase, Two-level)" : Subsystem  Variant=on  VariantControlMode=label  LabelModeActiveChoice=PWM
  Switch1 : Switch  Criteria=u2 > Threshold
  Unit Delay2 : UnitDelay  SampleTime=Tsc  HasFrameUpgradeWarning=on
  Zero vector : Constant  Value=zeros(6,1)  SampleTime=Ts
  G : Outport  VectorParamsAs1DForOutWhenUnconnected=off
  ModWave : Outport  Port=2  SampleTime=Tsc  VectorParamsAs1DForOutWhenUnconnected=off
  wires:
  theta/1 -> Inverse Park Transform/2
  vdqRef/1 -> Mux/1
  Mux/1 -> Inverse Park Transform/1
  Constant/1 -> Mux/2
  "PWM Generator (Three-phase, Two-level)"/2(ModWave) -> ModWave/1
  "PWM Generator (Three-phase, Two-level)"/1(g) -> Switch1/1
  PwmEnable/1 -> Unit Delay2/1
  Zero vector/1 -> Switch1/3
  Switch1/1 -> G/1
  Inverse Park Transform/1 -> "PWM Generator (Three-phase, Two-level)"/1(Vabc)
  Vdc/1 -> "PWM Generator (Three-phase, Two-level)"/2(vdc)
  Unit Delay2/1 -> Switch1/2

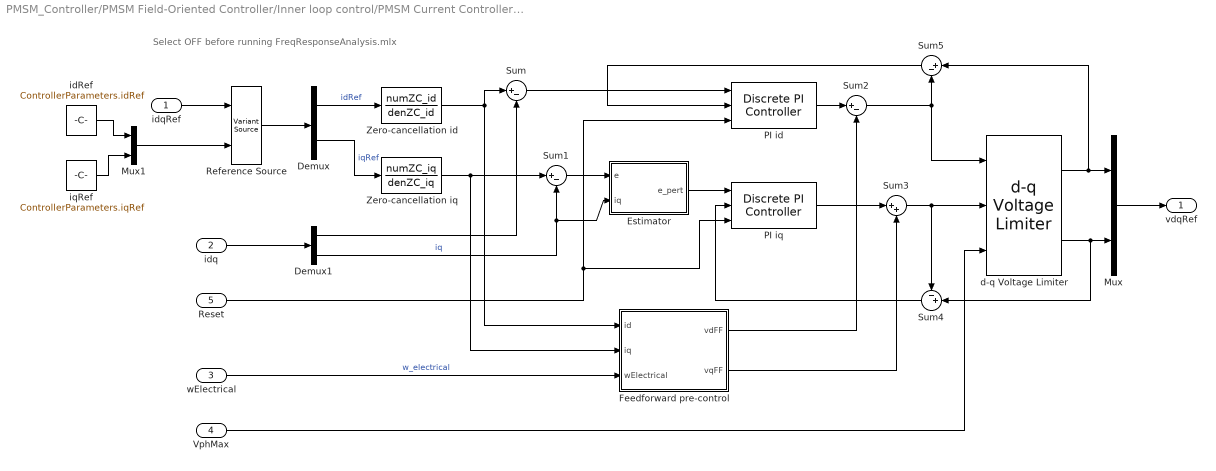
== system PMSM_Controller/PMSM Field-Oriented Controller/Inner loop control/PMSM Current Controller with Pre-Control ==
  note: Select OFF before running FreqResponseAnalysis.mlx
  idqRef : Inport  PortDimensions=2  SampleTime=Ts
  idq : Inport  Port=2  SampleTime=Ts
  wElectrical : Inport  Port=3  SampleTime=Ts
  VphMax : Inport  Port=4  SampleTime=Ts
  Reset : Inport  Port=5  SampleTime=Ts
  Demux : Demux  Outputs=2
  Demux1 : Demux  Outputs=2
  Estimator : Subsystem  Variant=on  VariantControlMode=label  LabelModeActiveChoice=OFF
  Feedforward pre-control : Subsystem
  Mux : Mux  Inputs=2
  Mux1 : Mux  Inputs=2
  PI id : eeDiscretePi/Discrete PI Controller  Kp=Kp_id  Ki=Ki_id  Kaw=Kaw_id  x0=0  Ts=Ts
      settings: SourceProductBaseCode=PS
  PI iq : eeDiscretePi/Discrete PI Controller  Kp=Kp_iq  Ki=Ki_iq  Kaw=Kaw_iq  x0=0  Ts=Ts
      settings: SourceProductBaseCode=PS
  Reference Source : VariantSource  VariantControlMode=label  LabelModeActiveChoice=OFF  ShowConditionOnBlock=on
  Sum{,1..2,5} (4 alike) : Sum  Inputs=|+-
  Sum3 : Sum  Inputs=|++
  Sum4 : Sum  Inputs=-+|
  Zero-cancellation id : DiscreteTransferFcn  Numerator=numZC_id  Denominator=denZC_id  SampleTime=Ts
  Zero-cancellation iq : DiscreteTransferFcn  Numerator=numZC_iq  Denominator=denZC_iq  SampleTime=Ts
  d-q Voltage Limiter : eeDqVoltageLimiter/d-q Voltage Limiter  AxisPrio=Q-axis  Ts=Ts
      settings: SourceProductBaseCode=PS
  idRef : Constant  Value=ControllerParameters.idRef
  iqRef : Constant  Value=ControllerParameters.iqRef
  vdqRef : Outport  VectorParamsAs1DForOutWhenUnconnected=off
  wires:
  Mux1/1 -> Reference Source/2
  Feedforward pre-control/2(vqFF) -> Sum3/2
  Feedforward pre-control/1(vdFF) -> Sum2/2
  PI iq/1 -> Sum3/1
  Sum1/1 -> Estimator/1(e)
  Estimator/1(e_pert) -> PI iq/1
  iqRef/1 -> Mux1/2
  idRef/1 -> Mux1/1
  Reference Source/1 -> Demux/1
  Sum2/1 -> d-q Voltage Limiter/1, Sum5/2
  Zero-cancellation id/1 -> Feedforward pre-control/1(id), Sum/1
  Mux/1 -> vdqRef/1
  Zero-cancellation iq/1 -> Sum1/1, Feedforward pre-control/2(iq)
  PI id/1 -> Sum2/1
  Sum/1 -> PI id/1
  d-q Voltage Limiter/1 -> Mux/1, Sum5/1
  Demux/1 -> Zero-cancellation id/1  "idRef"
  Sum3/1 -> d-q Voltage Limiter/2, Sum4/1
  Demux/2 -> Zero-cancellation iq/1  "iqRef"
  Sum4/1 -> PI iq/2
  d-q Voltage Limiter/2 -> Mux/2, Sum4/2
  Demux1/1 -> Sum/2
  Demux1/2 -> Estimator/2(iq), Sum1/2  "iq"
  Sum5/1 -> PI id/2
  idqRef/1 -> Reference Source/1
  idq/1 -> Demux1/1
  Reset/1 -> PI iq/3, PI id/3
  wElectrical/1 -> Feedforward pre-control/3(wElectrical)  "w_electrical"
  VphMax/1 -> d-q Voltage Limiter/3

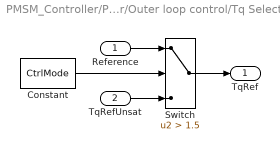
== system PMSM_Controller/PMSM Field-Oriented Controller/Outer loop control/Tq Selector ==
  Reference : Inport
  TqRefUnsat : Inport  Port=2
  Constant : Constant  Value=CtrlMode  SampleTime=Tsc
  Switch : Switch  Criteria=u2 > Threshold  Threshold=1.5
  TqRef : Outport  VectorParamsAs1DForOutWhenUnconnected=off
  wires:
  Switch/1 -> TqRef/1
  Constant/1 -> Switch/2
  TqRefUnsat/1 -> Switch/3
  Reference/1 -> Switch/1

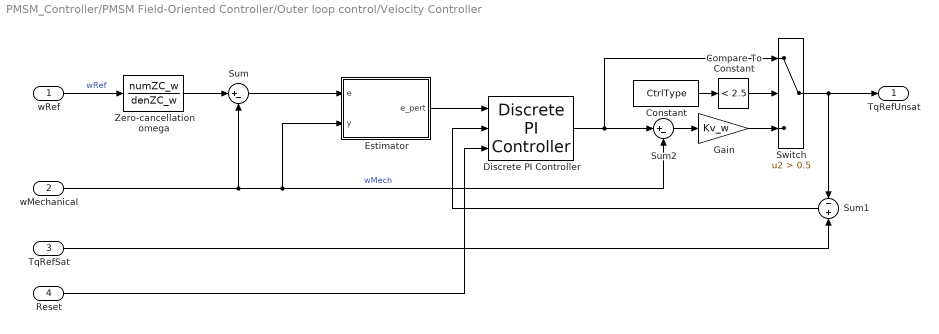
== system PMSM_Controller/PMSM Field-Oriented Controller/Outer loop control/Velocity Controller ==
  wRef : Inport  SampleTime=Ts
  wMechanical : Inport  Port=2  SampleTime=Ts
  TqRefSat : Inport  Port=3  SampleTime=Ts
  Reset : Inport  Port=4  SampleTime=Ts
  Compare To Constant : simulink/Logic and Bit Operations/Compare To Constant  relop=<  const=2.5  OutDataTypeStr=boolean
  Constant : Constant  Value=CtrlType  SampleTime=Ts
  Discrete PI Controller : eeDiscretePi/Discrete PI Controller  Kp=Kp_w  Ki=Ki_w  Kaw=Kaw_w  x0=0  Ts=Ts
      settings: SourceProductBaseCode=PS
  Estimator : Subsystem  Variant=on  VariantControlMode=label  LabelModeActiveChoice=OFF
  Gain : Gain  Gain=Kv_w
  Sum : Sum  Inputs=|+-
  Sum1 : Sum  Inputs=-+
  Sum2 : Sum  Inputs=|+-
  Switch : Switch  Criteria=u2 > Threshold  Threshold=0.5
  Zero-cancellation omega : DiscreteTransferFcn  Numerator=numZC_w  Denominator=denZC_w  SampleTime=Ts
  TqRefUnsat : Outport  VectorParamsAs1DForOutWhenUnconnected=off
  wires:
  Sum/1 -> Estimator/1(e)
  Estimator/1(e_pert) -> Discrete PI Controller/1
  Discrete PI Controller/1 -> Switch/1, Sum2/1
  Constant/1 -> Compare To Constant/1
  TqRefSat/1 -> Sum1/2
  Compare To Constant/1 -> Switch/2
  Zero-cancellation omega/1 -> Sum/1
  Reset/1 -> Discrete PI Controller/3
  Switch/1 -> Sum1/1, TqRefUnsat/1
  wRef/1 -> Zero-cancellation omega/1  "wRef"
  Sum1/1 -> Discrete PI Controller/2
  Sum2/1 -> Gain/1
  wMechanical/1 -> Estimator/2(y), Sum2/2, Sum/2  "wMech"
  Gain/1 -> Switch/3

== system PMSM_Controller/PMSM Field-Oriented Controller/PWM/PWM Generator (Three-phase, Two-level) ==
  Vabc : Inport
  vdc : Inport  Port=2
  PWM : eePwmGeneratorTwoLevel/PWM Generator (Three-phase, Two-level)  VariantControl=PWM  PWMMode=Continuous PWM (CPWM)  CPWMMode=SPWM: sinusoidal PWM  DPWMMode=60 DPWM: 60 degree discontinuous PWM  fsw=fsw  Ts=Ts
      settings: SourceProductBaseCode=PS
  g : Outport  VectorParamsAs1DForOutWhenUnconnected=off
  ModWave : Outport  Port=2  VectorParamsAs1DForOutWhenUnconnected=off

== system PMSM_Controller/PMSM Field-Oriented Controller/Inner loop control/PMSM Current Controller with Pre-Control/Estimator ==
  e : Inport
  iq : Inport  Port=2
  OFF : Subsystem  VariantControl=OFF
  ON : Subsystem  VariantControl=ON
  e_pert : Outport

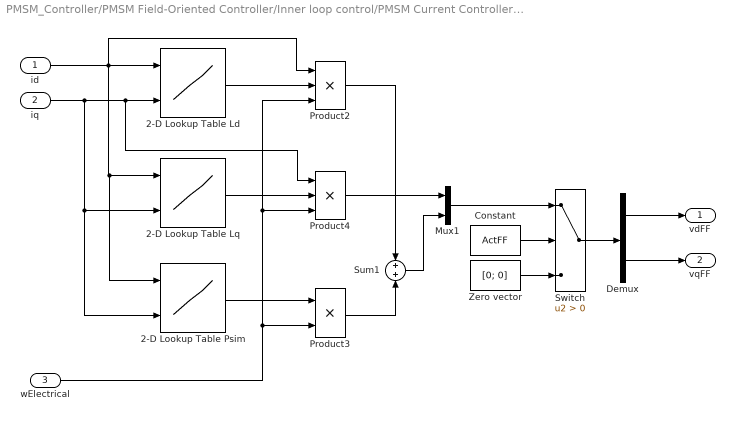
== system PMSM_Controller/PMSM Field-Oriented Controller/Inner loop control/PMSM Current Controller with Pre-Control/Feedforward pre-control ==
  id : Inport
  iq : Inport  Port=2
  wElectrical : Inport  Port=3
  2-D Lookup Table Ld : Lookup_n-D  BreakpointsForDimension1=idVect  BreakpointsForDimension2=iqVect  Table=LdMatrix  ExtrapMethod=Clip  UseLastTableValue=on  InternalRulePriority=Speed  RndMeth=Simplest  InputSameDT=on
      settings: InputPortMap=u0,u1
  2-D Lookup Table Lq : Lookup_n-D  BreakpointsForDimension1=idVect  BreakpointsForDimension2=iqVect  Table=LqMatrix  ExtrapMethod=Clip  InternalRulePriority=Speed  RndMeth=Simplest  InputSameDT=on
      settings: InputPortMap=u0,u1
  2-D Lookup Table Psim : Lookup_n-D  BreakpointsForDimension1=idVect  BreakpointsForDimension2=iqVect  Table=psimMatrix  ExtrapMethod=Clip  InternalRulePriority=Speed  RndMeth=Simplest  InputSameDT=on
      settings: InputPortMap=u0,u1
  Constant : Constant  Value=ActFF  SampleTime=Ts
  Demux : Demux  Outputs=2
  Mux1 : Mux  Inputs=2
  Product2 : Product  Inputs=3
  Product3 : Product
  Product4 : Product  Inputs=3
  Sum1 : Sum
  Switch : Switch  Criteria=u2 > Threshold
  Zero vector : Constant  Value=[0; 0]  SampleTime=Ts
  vdFF : Outport  VectorParamsAs1DForOutWhenUnconnected=off
  vqFF : Outport  Port=2  VectorParamsAs1DForOutWhenUnconnected=off
  wires:
  Product3/1 -> Sum1/2
  2-D Lookup Table Lq/1 -> Product4/2
  Constant/1 -> Switch/2
  Switch/1 -> Demux/1
  Demux/1 -> vdFF/1
  Demux/2 -> vqFF/1
  2-D Lookup Table Psim/1 -> Product3/1
  Zero vector/1 -> Switch/3
  Sum1/1 -> Mux1/2
  2-D Lookup Table Ld/1 -> Product2/2
  iq/1 -> Product4/1, 2-D Lookup Table Ld/2, 2-D Lookup Table Lq/2, 2-D Lookup Table Psim/2
  id/1 -> Product2/1, 2-D Lookup Table Psim/1, 2-D Lookup Table Lq/1, 2-D Lookup Table Ld/1
  Product4/1 -> Mux1/1
  Mux1/1 -> Switch/1
  wElectrical/1 -> Product3/2, Product4/3, Product2/3
  Product2/1 -> Sum1/1

== system PMSM_Controller/PMSM Field-Oriented Controller/Outer loop control/Velocity Controller/Estimator ==
  e : Inport
  y : Inport  Port=2
  OFF : Subsystem  VariantControl=OFF
  ON : Subsystem  VariantControl=ON
  e_pert : Outport

== system PMSM_Controller/PMSM Field-Oriented Controller/Inner loop control/PMSM Current Controller with Pre-Control/Estimator/OFF ==
  e : Inport
  e_pert : Outport
  wires:
  e/1 -> e_pert/1

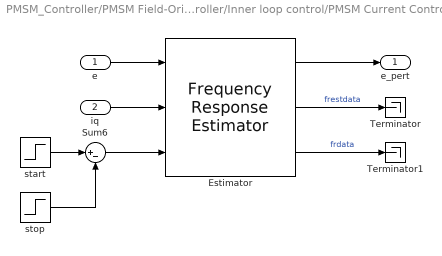
== system PMSM_Controller/PMSM Field-Oriented Controller/Inner loop control/PMSM Current Controller with Pre-Control/Estimator/ON ==
  e : Inport
  iq : Inport  Port=2
  Estimator : slctrlblks/Frequency Response Estimator  DiscreteTs=Ts  OutputMode=control action + perturbation  BlockDataType=double  SineSource=Block parameters  Frequencies=logspace(2,4,10)  FreqUnits=rad/s  Amplitudes=100  NumOfFreq=3  ExperimentMode=Sinestream  NumOfSetPeriod=2  NumOfEstPeriod=3  NumOfSlowestPeriod=3  EstimationMode=Online  UseBodePlot=off  BaselinePlant=[]  PlotRefreshFactor=100  BodePlotChoice=VariantNull  ExperimentChoice=VariantSS  OutputChoice=VariantCandD
      settings: SourceProductBaseCode=SD
  Sum6 : Sum  Inputs=|+-
  Terminator : Terminator
  Terminator1 : Terminator
  start : Step  Time=0.1  SampleTime=0
  stop : Step  Time=0.9  SampleTime=0
  e_pert : Outport
  wires:
  Estimator/3 -> Terminator1/1  "frdata"
  stop/1 -> Sum6/2
  Estimator/2 -> Terminator/1  "frestdata"
  iq/1 -> Estimator/2
  e/1 -> Estimator/1
  Sum6/1 -> Estimator/3
  Estimator/1 -> e_pert/1
  start/1 -> Sum6/1

== system PMSM_Controller/PMSM Field-Oriented Controller/Outer loop control/Velocity Controller/Estimator/OFF ==
  e : Inport
  e_pert : Outport
  wires:
  e/1 -> e_pert/1

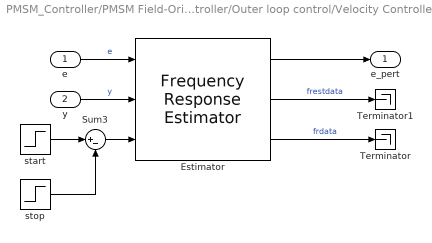
== system PMSM_Controller/PMSM Field-Oriented Controller/Outer loop control/Velocity Controller/Estimator/ON ==
  e : Inport
  y : Inport  Port=2
  Estimator : slctrlblks/Frequency Response Estimator  DiscreteTs=Ts  OutputMode=control action + perturbation  BlockDataType=double  SineSource=Block parameters  Frequencies=logspace(3,4,5)  FreqUnits=rad/s  Amplitudes=1  NumOfFreq=3  ExperimentMode=Sinestream  NumOfSetPeriod=3  NumOfEstPeriod=15  NumOfSlowestPeriod=3  EstimationMode=Online  UseBodePlot=on  BaselinePlant=[]  PlotRefreshFactor=100  BodePlotChoice=VariantBode  ExperimentChoice=VariantSS  OutputChoice=VariantCandD
      settings: SourceProductBaseCode=SD
  Sum3 : Sum  Inputs=|+-
  Terminator : Terminator
  Terminator1 : Terminator
  start : Step  Time=0.2  SampleTime=0
  stop : Step  Time=0.45  SampleTime=0
  e_pert : Outport
  wires:
  Estimator/1 -> e_pert/1
  start/1 -> Sum3/1
  Estimator/3 -> Terminator/1  "frdata"
  Estimator/2 -> Terminator1/1  "frestdata"
  y/1 -> Estimator/2  "y"
  e/1 -> Estimator/1  "e"
  Sum3/1 -> Estimator/3
  stop/1 -> Sum3/2
